simulink model "Model"  (R2022b)
settings: Solver=VariableStepAuto  StartTime=0.0  StopTime=10.0  RelTol=1e-3
values from neighbouring files (symbols this model uses):
  tau = 0.084    [ModeloMotor_v1.m]
undefined symbols (not defined in the file or in its folder): Fx_idq, id, iq
settings Model: Creator=Javier  LastModifiedBy=ramuj
settings DebuggingCC: UnconnectedInputMsg=warning  UnconnectedOutputMsg=warning  UnconnectedLineMsg=warning
settings ModelReferenceCC: EnableRefExpFcnMdlSchedulingChecks=on
settings RTWCC: DLArmComputeVersion=19.05

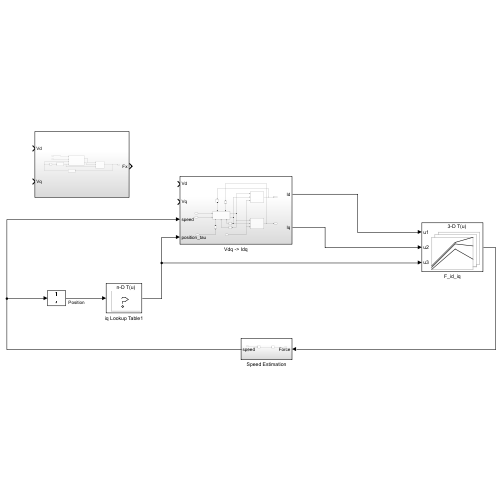
[thumbnail: Simulink's stored preview of the top-level diagram]
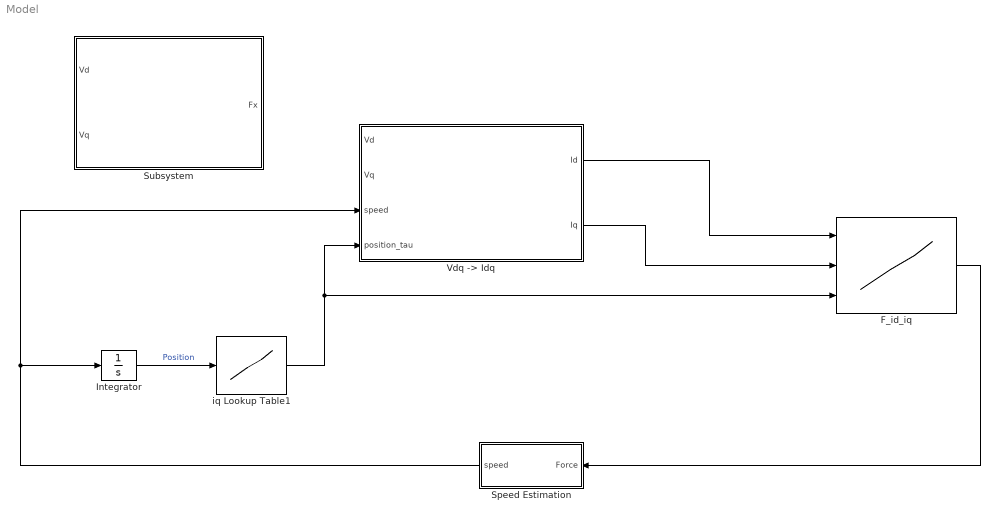
== system Model ==
  F_id_iq : Lookup_n-D  NumberOfTableDimensions=3  BreakpointsForDimension3=[5, 7]  Table=reshape(repmat([4 5 6;16 19 20;10 18 23],1,2),[3,3,2])  InternalRulePriority=Speed  RndMeth=Simplest
      settings: InputPortMap=u0,u1,u2
  Integrator : Integrator
  Speed Estimation : Subsystem
  Subsystem : Subsystem
  "Vdq -> Idq" : Subsystem
  iq Lookup Table1 : Lookup_n-D  NumberOfTableDimensions=1  BreakpointsForDimension3=[5, 7]  Table=reshape(repmat([4 5 6;16 19 20;10 18 23],1,2),[3,3,2])  InternalRulePriority=Speed  RndMeth=Simplest
  wires:
  Integrator/1 -> iq Lookup Table1/1  "Position"
  iq Lookup Table1/1 -> F_id_iq/3, "Vdq -> Idq"/4(position_tau)
  Speed Estimation/1(speed) -> Integrator/1, "Vdq -> Idq"/3(speed)
  "Vdq -> Idq"/1(Id) -> F_id_iq/1
  "Vdq -> Idq"/2(Iq) -> F_id_iq/2
  F_id_iq/1 -> Speed Estimation/1(Force)

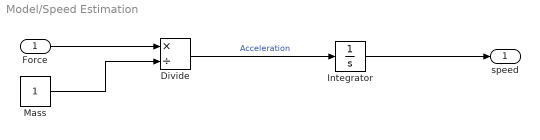
== system Model/Speed Estimation ==
  Force : Inport
  Divide : Product  Inputs=*/
  Integrator : Integrator
  Mass : Constant
  speed : Outport
  wires:
  Force/1 -> Divide/1
  Mass/1 -> Divide/2
  Divide/1 -> Integrator/1  "Acceleration"
  Integrator/1 -> speed/1

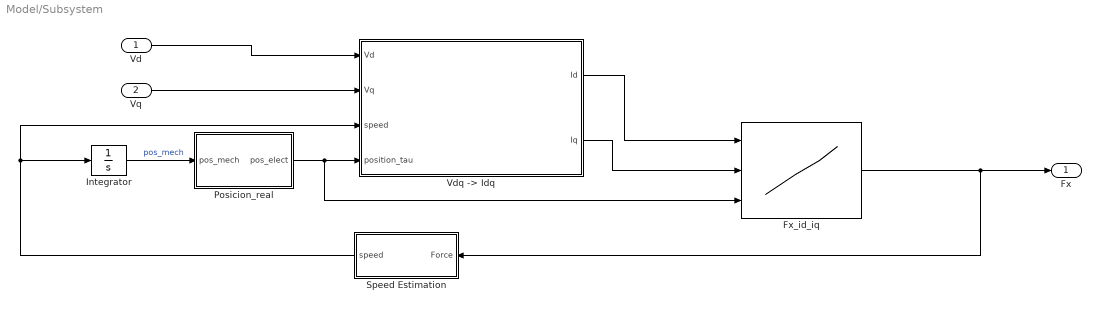
== system Model/Subsystem ==
  Vd : Inport
  Vq : Inport  Port=2
  Fx_id_iq : Lookup_n-D  NumberOfTableDimensions=3  BreakpointsForDimension1=id  BreakpointsForDimension2=iq  BreakpointsForDimension3=angle  Table=Fx_idq  InternalRulePriority=Speed  RndMeth=Simplest
      settings: InputPortMap=u0,u1,u2
  Integrator : Integrator
  Posicion_real : Subsystem
  Speed Estimation : Subsystem
  "Vdq -> Idq" : Subsystem
  Fx : Outport
  wires:
  Speed Estimation/1(speed) -> Integrator/1, "Vdq -> Idq"/3(speed)
  Posicion_real/1(pos_elect) -> Fx_id_iq/3, "Vdq -> Idq"/4(position_tau)
  "Vdq -> Idq"/2(Iq) -> Fx_id_iq/2
  Integrator/1 -> Posicion_real/1(pos_mech)  "pos_mech"
  "Vdq -> Idq"/1(Id) -> Fx_id_iq/1
  Vq/1 -> "Vdq -> Idq"/2(Vq)
  Vd/1 -> "Vdq -> Idq"/1(Vd)
  Fx_id_iq/1 -> Fx/1, Speed Estimation/1(Force)

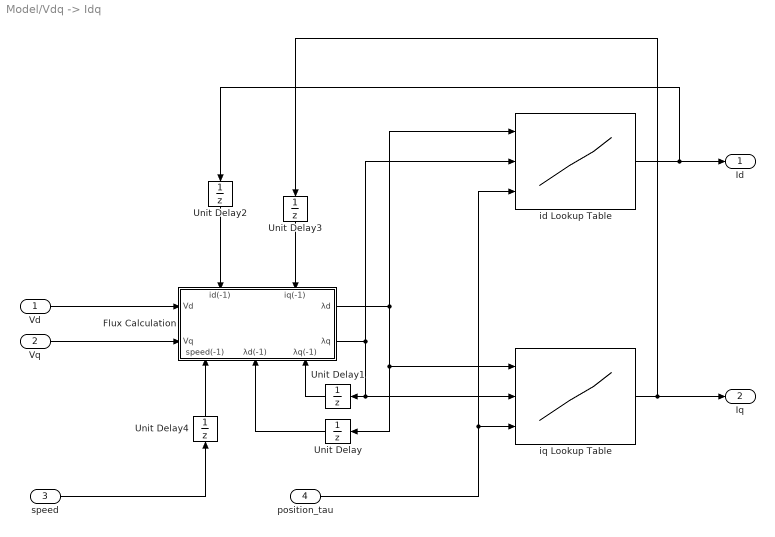
== system Model/Vdq -> Idq ==
  Vd : Inport
  Vq : Inport  Port=2
  speed : Inport  Port=3
  position_tau : Inport  Port=4
  Flux Calculation : Subsystem
      settings: PortSchema="{\"entries\":[{\"content\":{\"sides\":[{\"content\":{\"connectorIds\":[\"In1\",\"In2\"]},\"type\":\"ConnectorPlacement.EquallySpacedRectSide\",\"uuid\":\"ad8eb314-33c9-4fb6-897d-d070f38f086b\"},{\"content\":{\"connectorIds\":[\"Out1\",\"Out2\"],\"side\":\"RIGHT\"},\"type\":\"ConnectorPlacement.EquallySpacedRectSide\",\"uuid\":\"d1d8c5ab-4de0-4214-bbc7-93acdad91b9d\"},{\"content\":{\"connectorIds\":[\"In3\",\"In4\"],\"side\":\"TOP\"},\"type\":\"ConnectorPlacement.EquallySpacedRectSide\",\"uuid\":\"c81f1c6d-9cfa-4c7d-8c6d-bc8ee29731ad\"},{\"content\":{\"connectorIds\":[\"In5\",\"In6\",\"In7\"],\"side\":\"BOTTOM\"},\"type\":\"ConnectorPlacement.EquallySpacedRectSide\",\"uuid\":\"f872afb0-75ae-4dbb-8707-51300132d239\"}]},\"type\":\"ConnectorPlacement.EquallySpacedConnector\",\"uuid\":\"dd7b761d-a9cf-4410-8aff-8d775c3295c0\"}],\"packageUris\":[\"http://schema.mathworks.com/mf0/Connector/R2020b\"],\"version\":\"1.0\"}"
  Unit Delay{,1..4} (5 alike) : UnitDelay  SampleTime=-1  HasFrameUpgradeWarning=on
  id Lookup Table : Lookup_n-D  NumberOfTableDimensions=3  BreakpointsForDimension3=[5, 7]  Table=reshape(repmat([4 5 6;16 19 20;10 18 23],1,2),[3,3,2])  InternalRulePriority=Speed  RndMeth=Simplest
      settings: InputPortMap=u0,u1,u2
  iq Lookup Table : Lookup_n-D  NumberOfTableDimensions=3  BreakpointsForDimension3=[5, 7]  Table=reshape(repmat([4 5 6;16 19 20;10 18 23],1,2),[3,3,2])  InternalRulePriority=Speed  RndMeth=Simplest
      settings: InputPortMap=u0,u1,u2
  Id : Outport
  Iq : Outport  Port=2
  wires:
  Vd/1 -> Flux Calculation/1(Vd)
  Vq/1 -> Flux Calculation/2(Vq)
  Flux Calculation/1(λd) -> Unit Delay/1, iq Lookup Table/1, id Lookup Table/1
  Unit Delay/1 -> Flux Calculation/6(λd(-1))
  Flux Calculation/2(λq) -> Unit Delay1/1, iq Lookup Table/2, id Lookup Table/2
  Unit Delay1/1 -> Flux Calculation/7(λq(-1))
  Unit Delay2/1 -> Flux Calculation/3(id(-1))
  Unit Delay3/1 -> Flux Calculation/4(iq(-1))
  Unit Delay4/1 -> Flux Calculation/5(speed(-1))
  speed/1 -> Unit Delay4/1
  id Lookup Table/1 -> Unit Delay2/1, Id/1
  iq Lookup Table/1 -> Iq/1, Unit Delay3/1
  position_tau/1 -> iq Lookup Table/3, id Lookup Table/3

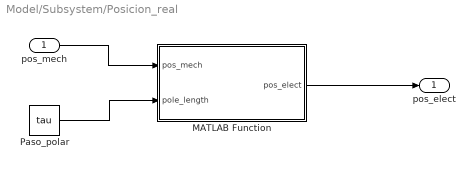
== system Model/Subsystem/Posicion_real ==
  pos_mech : Inport
  MATLAB Function : MATLAB Function  TreatAsAtomicUnit=on
  Paso_polar : Constant  Value=tau
  pos_elect : Outport
  wires:
  MATLAB Function/1(pos_elect) -> pos_elect/1
  pos_mech/1 -> MATLAB Function/1(pos_mech)
  Paso_polar/1 -> MATLAB Function/2(pole_length)

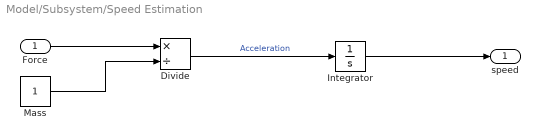
== system Model/Subsystem/Speed Estimation ==
  Force : Inport
  Divide : Product  Inputs=*/
  Integrator : Integrator
  Mass : Constant
  speed : Outport
  wires:
  Force/1 -> Divide/1
  Mass/1 -> Divide/2
  Divide/1 -> Integrator/1  "Acceleration"
  Integrator/1 -> speed/1

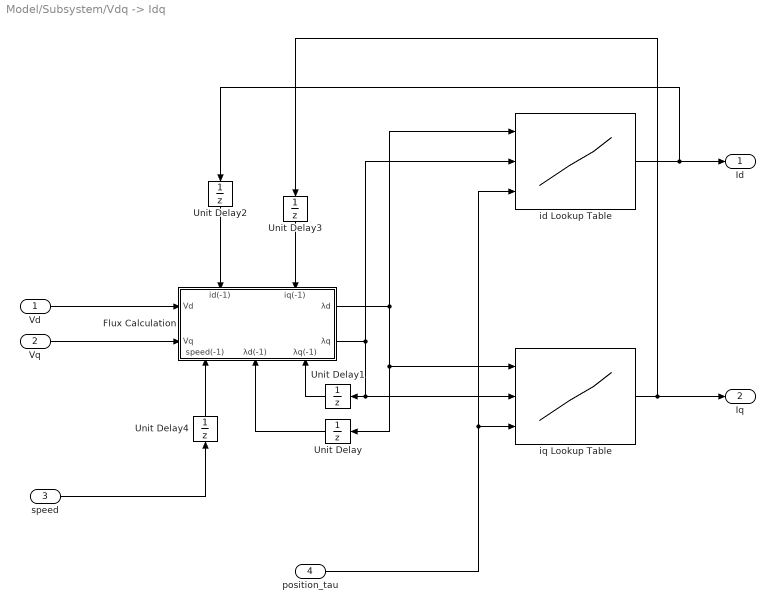
== system Model/Subsystem/Vdq -> Idq ==
  Vd : Inport
  Vq : Inport  Port=2
  speed : Inport  Port=3
  position_tau : Inport  Port=4
  Flux Calculation : Subsystem
      settings: PortSchema="{\"entries\":[{\"content\":{\"sides\":[{\"content\":{\"connectorIds\":[\"In1\",\"In2\"]},\"type\":\"ConnectorPlacement.EquallySpacedRectSide\",\"uuid\":\"ad8eb314-33c9-4fb6-897d-d070f38f086b\"},{\"content\":{\"connectorIds\":[\"Out1\",\"Out2\"],\"side\":\"RIGHT\"},\"type\":\"ConnectorPlacement.EquallySpacedRectSide\",\"uuid\":\"d1d8c5ab-4de0-4214-bbc7-93acdad91b9d\"},{\"content\":{\"connectorIds\":[\"In3\",\"In4\"],\"side\":\"TOP\"},\"type\":\"ConnectorPlacement.EquallySpacedRectSide\",\"uuid\":\"c81f1c6d-9cfa-4c7d-8c6d-bc8ee29731ad\"},{\"content\":{\"connectorIds\":[\"In5\",\"In6\",\"In7\"],\"side\":\"BOTTOM\"},\"type\":\"ConnectorPlacement.EquallySpacedRectSide\",\"uuid\":\"f872afb0-75ae-4dbb-8707-51300132d239\"}]},\"type\":\"ConnectorPlacement.EquallySpacedConnector\",\"uuid\":\"dd7b761d-a9cf-4410-8aff-8d775c3295c0\"}],\"packageUris\":[\"http://schema.mathworks.com/mf0/Connector/R2020b\"],\"version\":\"1.0\"}"
  Unit Delay{,1..4} (5 alike) : UnitDelay  SampleTime=-1  HasFrameUpgradeWarning=on
  id Lookup Table : Lookup_n-D  NumberOfTableDimensions=3  BreakpointsForDimension3=[5, 7]  Table=reshape(repmat([4 5 6;16 19 20;10 18 23],1,2),[3,3,2])  InternalRulePriority=Speed  RndMeth=Simplest
      settings: InputPortMap=u0,u1,u2
  iq Lookup Table : Lookup_n-D  NumberOfTableDimensions=3  BreakpointsForDimension3=[5, 7]  Table=reshape(repmat([4 5 6;16 19 20;10 18 23],1,2),[3,3,2])  InternalRulePriority=Speed  RndMeth=Simplest
      settings: InputPortMap=u0,u1,u2
  Id : Outport
  Iq : Outport  Port=2
  wires:
  Vd/1 -> Flux Calculation/1(Vd)
  Vq/1 -> Flux Calculation/2(Vq)
  Flux Calculation/1(λd) -> Unit Delay/1, iq Lookup Table/1, id Lookup Table/1
  Unit Delay/1 -> Flux Calculation/6(λd(-1))
  Flux Calculation/2(λq) -> Unit Delay1/1, iq Lookup Table/2, id Lookup Table/2
  Unit Delay1/1 -> Flux Calculation/7(λq(-1))
  Unit Delay2/1 -> Flux Calculation/3(id(-1))
  Unit Delay3/1 -> Flux Calculation/4(iq(-1))
  Unit Delay4/1 -> Flux Calculation/5(speed(-1))
  speed/1 -> Unit Delay4/1
  id Lookup Table/1 -> Unit Delay2/1, Id/1
  iq Lookup Table/1 -> Iq/1, Unit Delay3/1
  position_tau/1 -> iq Lookup Table/3, id Lookup Table/3

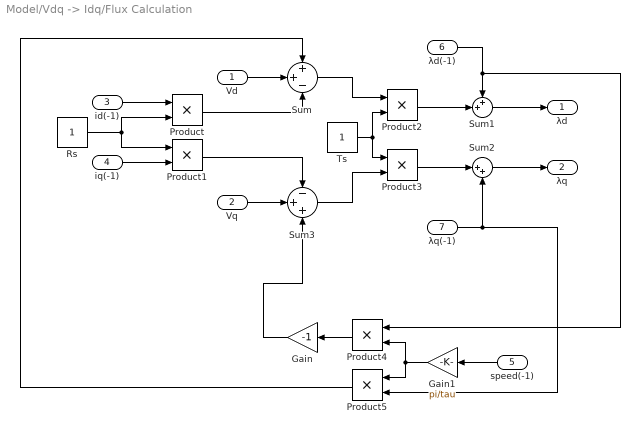
== system Model/Vdq -> Idq/Flux Calculation ==
  Vd : Inport
  Vq : Inport  Port=2
  id(-1) : Inport  Port=3
  iq(-1) : Inport  Port=4
  speed(-1) : Inport  Port=5
  λd(-1) : Inport  Port=6
  λq(-1) : Inport  Port=7
  Gain : Gain  Gain=-1
  Gain1 : Gain  Gain=pi/tau
  Product{,1..5} (6 alike) : Product
  Rs : Constant
  Sum : Sum  Inputs=++-
  Sum1 : Sum  Inputs=++|
  Sum2 : Sum  Inputs=|++
  Sum3 : Sum  Inputs=-++
  Ts : Constant
  λd : Outport
  λq : Outport  Port=2
  wires:
  Rs/1 -> Product1/1, Product/2
  id(-1)/1 -> Product/1
  iq(-1)/1 -> Product1/2
  Product/1 -> Sum/3
  Vd/1 -> Sum/2
  Sum/1 -> Product2/1
  Ts/1 -> Product3/1, Product2/2
  Product2/1 -> Sum1/2
  λq(-1)/1 -> Sum2/2, Product5/2
  λd(-1)/1 -> Product4/1, Sum1/1
  Sum1/1 -> λd/1
  Sum2/1 -> λq/1
  Product3/1 -> Sum2/1
  Product1/1 -> Sum3/1
  Product4/1 -> Gain/1
  Gain/1 -> Sum3/3
  Vq/1 -> Sum3/2
  Sum3/1 -> Product3/2
  Product5/1 -> Sum/1
  speed(-1)/1 -> Gain1/1
  Gain1/1 -> Product5/1, Product4/2

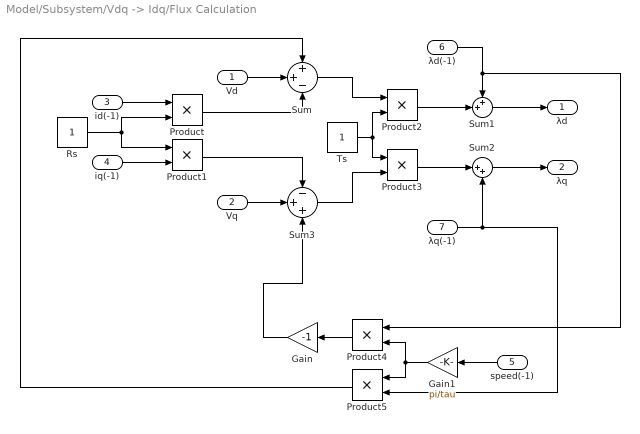
== system Model/Subsystem/Vdq -> Idq/Flux Calculation ==
  Vd : Inport
  Vq : Inport  Port=2
  id(-1) : Inport  Port=3
  iq(-1) : Inport  Port=4
  speed(-1) : Inport  Port=5
  λd(-1) : Inport  Port=6
  λq(-1) : Inport  Port=7
  Gain : Gain  Gain=-1
  Gain1 : Gain  Gain=pi/tau
  Product{,1..5} (6 alike) : Product
  Rs : Constant
  Sum : Sum  Inputs=++-
  Sum1 : Sum  Inputs=++|
  Sum2 : Sum  Inputs=|++
  Sum3 : Sum  Inputs=-++
  Ts : Constant
  λd : Outport
  λq : Outport  Port=2
  wires:
  Rs/1 -> Product1/1, Product/2
  id(-1)/1 -> Product/1
  iq(-1)/1 -> Product1/2
  Product/1 -> Sum/3
  Vd/1 -> Sum/2
  Sum/1 -> Product2/1
  Ts/1 -> Product3/1, Product2/2
  Product2/1 -> Sum1/2
  λq(-1)/1 -> Sum2/2, Product5/2
  λd(-1)/1 -> Product4/1, Sum1/1
  Sum1/1 -> λd/1
  Sum2/1 -> λq/1
  Product3/1 -> Sum2/1
  Product1/1 -> Sum3/1
  Product4/1 -> Gain/1
  Gain/1 -> Sum3/3
  Vq/1 -> Sum3/2
  Sum3/1 -> Product3/2
  Product5/1 -> Sum/1
  speed(-1)/1 -> Gain1/1
  Gain1/1 -> Product5/1, Product4/2

== matlab function Model/Subsystem/Posicion_real/MATLAB Function ==
  data: pos_mech input; pos_elect output; pole_length input
function pos_elect = fcn(pos_mech,pole_length)

k=fix(pos_mech/pole_length);
pos_elect=pos_mech-k*pole_length;
